simulink subsystem "InverterMotor"  (R2023b)
settings: Solver=VariableStepAuto  StartTime=0.0  StopTime=10.0  RelTol=1e-3
undefined symbols (not defined in the file): F, J, Ld, Lq, NPoles, Tf, TMotorMax, tSimMoCo
libraries: autolibpmsminterior x1, autolibinverter x1
settings Model: Creator=Elio  LastModifiedBy=Elio

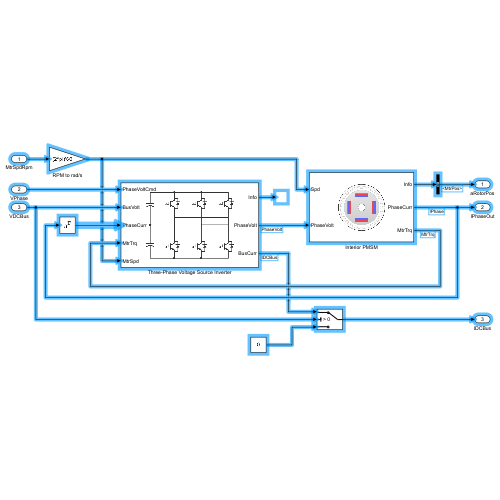
[thumbnail: Simulink's stored preview of the top-level diagram]
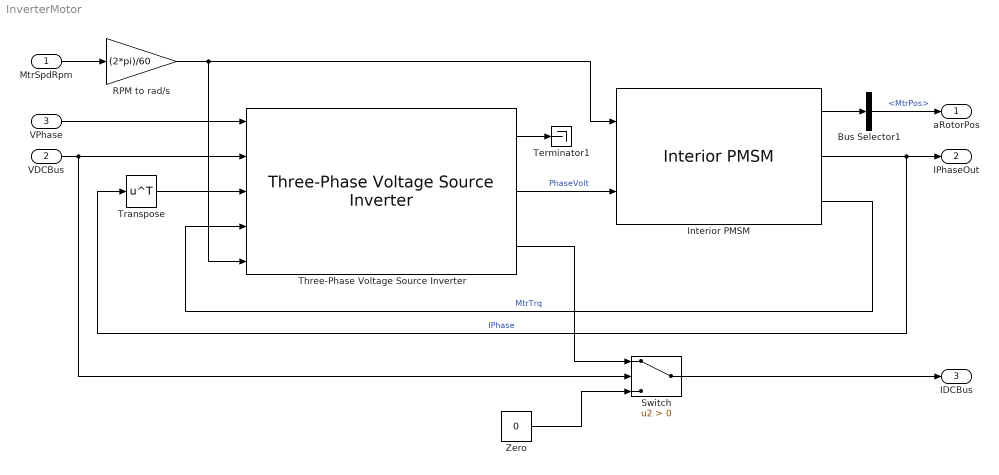
== system InverterMotor ==
  MtrSpdRpm : Inport
  VDCBus : Inport  Port=2
  VPhase : Inport  Port=3
  Bus Selector1 : BusSelector  OutputSignals=MtrPos
  Interior PMSM : autolibpmsminterior/Interior PMSM  port_config=Speed  sim_type=Discrete  Ts=tSimMoCo  FilePath=interiorpmsm_motordata.m  P=NPoles  Rs=Rs  Ldq=[Ld Lq]  KConstText=Permanent flux linkage constant (lambda_pm):  lambda_pm=PMFluxLinkage  Ke=Ke  mechanical=[J, F, Tf]  idq0=[0 0]  theta_init=0  omega_init=0  KConst=PMFluxLinkage  lambda_pm_calc=PMFluxLinkage  Kt=1.323  RefBlkName='autolibpmsminterior/Interior PMSM'  aMode=1
      settings: LibrarySourceBlock=autolibemachines/Interior PMSM
  RPM to rad/s : Gain  Gain=(2*pi)/60
  Switch : Switch  Criteria=u2 > Threshold  SaturateOnIntegerOverflow=off  InputSameDT=off
  Terminator1 : Terminator
  Three-Phase Voltage Source Inverter : autolibinverter/Three-Phase Voltage Source Inverter  InvrtrTmpInpEnbl=off  enable_hdl=off  model_type=Commanded phase voltage  fs=10000  w_eff_bp=w_eff_bp  n1=128  T_eff_bp=[-TMotorMax -TMotorMax/2 0 TMotorMax/2 TMotorMax]  Temp_eff_bp=[213.15 293.15 373.15]  n2=128  ploss_table=ploss_table  ploss_table_3d=cat(3,0.95*[1 0.999 0.989 0.997 0.996;0.995 0.994 0.993 0.992 0.991;0.990 0.989 0.988 0.987 0.986;0.985 0.984 0.983 0.982 0.981;0.980 0.979 0.978 0.977 0.976],[1 0.999 0.989 0.997 0.996;0.995 0.994 0.993 0.992 0.991;0.990 0.989 0.988 0.987 0.986;0.985 0.984 0.983 0.982 0.981;0.980 0.979 0.978 0.977 0.976],0.92*[1 0.999 0.989 0.997 0.996;0.995 0.994 0.993 0.992 0.991;0.990 0.989 0.988 0.987 0.986;0.985 0.984 0.983 0.982 0.981;0.980 0.979 0.978 0.977 0.976])  preExtrapFlag=off  u1max=1000  u1min=-1000  u2max=200  u2min=-200  intPrec=23  RefBlkName='autolibmappedmotor/Mapped Motor'  CalLossMapData={}  CalLossWithTempMapData={}
      settings: LibrarySourceBlock=autolibemachines/Three-Phase Voltage Source Inverter
  Transpose : Math  Operator=transpose
  Zero : Constant  Value=0  OutDataTypeStr=Inherit: Inherit via back propagation
  aRotorPos : Outport
  IPhaseOut : Outport  Port=2
  IDCBus : Outport  Port=3
  wires:
  Interior PMSM/2 -> Transpose/1, IPhaseOut/1  "IPhase"
  Interior PMSM/3 -> Three-Phase Voltage Source Inverter/4  "MtrTrq"
  Three-Phase Voltage Source Inverter/3 -> Switch/1
  Bus Selector1/1 -> aRotorPos/1  "<MtrPos>"
  VDCBus/1 -> Switch/2, Three-Phase Voltage Source Inverter/2
  Switch/1 -> IDCBus/1
  Three-Phase Voltage Source Inverter/1 -> Terminator1/1
  Zero/1 -> Switch/3
  MtrSpdRpm/1 -> RPM to rad/s/1
  VPhase/1 -> Three-Phase Voltage Source Inverter/1
  Interior PMSM/1 -> Bus Selector1/1
  RPM to rad/s/1 -> Three-Phase Voltage Source Inverter/5, Interior PMSM/1
  Three-Phase Voltage Source Inverter/2 -> Interior PMSM/2  "PhaseVolt"
  Transpose/1 -> Three-Phase Voltage Source Inverter/3
